simulink model "state_space_all_reduce_uio"  (R2018a)
settings: Solver=FixedStepAuto  StartTime=0.0  StopTime=3  FixedStep=tm  MaxStep=1e-4  RelTol=1e-5  AbsTol=1e-5
InitFcn:
  | SimulinkInit_linea_transmision
values from neighbouring files (symbols this model uses):
  b = 4.91    [SimulinkInit_linea_transmision.m]
  C = 1    [SimulinkInit_linea_transmision.m]
  C1 = 22e-6    (= 2.2e-05)    [SimulinkInit_linea_transmision.m]
  C2 = 22e-6    (= 2.2e-05)    [SimulinkInit_linea_transmision.m]
  C3 = 610e-6    (= 0.00061)    [SimulinkInit_linea_transmision.m]
  Cl = 20000e-6    (= 0.02)    [SimulinkInit_linea_transmision.m]
  Jd = 0.3    [SimulinkInit_linea_transmision.m]
  K = 25    [SimulinkInit_linea_transmision.m]    (also in uio_linear.m = K1+E*H)
  K1 = 9.66    [SimulinkInit_linea_transmision.m]    (also in uio_linear.m = K1')
  K11 = 0.8    [SimulinkInit_linea_transmision.m]
  K1d = 1.15    [SimulinkInit_linea_transmision.m]
  K2 = 6.97    [SimulinkInit_linea_transmision.m]
  K22 = 0.2    [SimulinkInit_linea_transmision.m]
  K2d = 1    [SimulinkInit_linea_transmision.m]
  K3 = 31.8    [SimulinkInit_linea_transmision.m]
  K33 = 0.23    [SimulinkInit_linea_transmision.m]
  K3d = 1    [SimulinkInit_linea_transmision.m]
  K4 = 15.1    [SimulinkInit_linea_transmision.m]
  Kd = 0.02    [SimulinkInit_linea_transmision.m]
  Kdc = 0.02    [SimulinkInit_linea_transmision.m]
  Kf = 1    [SimulinkInit_linea_transmision.m]
  Kh = 1.2    [SimulinkInit_linea_transmision.m]
  Ks = 21.5    [SimulinkInit_linea_transmision.m]
  Ksc = 3    [SimulinkInit_linea_transmision.m]
  Kv = 1    [SimulinkInit_linea_transmision.m]
  L = 5.2    [SimulinkInit_linea_transmision.m]
  L1 = 40e-3    (= 0.04)    [SimulinkInit_linea_transmision.m]
  L2 = 30e-3    (= 0.03)    [SimulinkInit_linea_transmision.m]
  L3 = 5e-3    (= 0.005)    [SimulinkInit_linea_transmision.m]
  L4 = 35e-6    (= 3.5e-05)    [SimulinkInit_linea_transmision.m]
  L5 = 22e-6    (= 2.2e-05)    [SimulinkInit_linea_transmision.m]
  L6 = 10e-6    (= 1e-05)    [SimulinkInit_linea_transmision.m]
  Pd = 0.1    [SimulinkInit_linea_transmision.m]
  R = 10    [SimulinkInit_linea_transmision.m]
  R1 = 0.1    [SimulinkInit_linea_transmision.m]
  R2 = 0.2    [SimulinkInit_linea_transmision.m]
  R3 = 1e-3    (= 0.001)    [SimulinkInit_linea_transmision.m]
  R4 = 0.005    [SimulinkInit_linea_transmision.m]
  R5 = 0.0012    [SimulinkInit_linea_transmision.m]
  R6 = 0.001    [SimulinkInit_linea_transmision.m]
  RL = 10    [SimulinkInit_linea_transmision.m]
  Sbin = 13.8    [SimulinkInit_linea_transmision.m]
  Svin = 2.91    [SimulinkInit_linea_transmision.m]
  T1 = 0.4    [SimulinkInit_linea_transmision.m]
  T2 = 1    [SimulinkInit_linea_transmision.m]
  T3 = 15    [SimulinkInit_linea_transmision.m]
  T4 = 2.5    [SimulinkInit_linea_transmision.m]
  Tao1d = 0.5    [SimulinkInit_linea_transmision.m]
  Tao2d = 0.125    [SimulinkInit_linea_transmision.m]
  Tcd = 0.2    [SimulinkInit_linea_transmision.m]
  Tcr = 0.01    [SimulinkInit_linea_transmision.m]
  Tf = 0.04    [SimulinkInit_linea_transmision.m]
  Tr = 950    [SimulinkInit_linea_transmision.m]
  Tt = 450    [SimulinkInit_linea_transmision.m]
  Ttd = 0.04    [SimulinkInit_linea_transmision.m]
  Tv = 0.05    [SimulinkInit_linea_transmision.m]
  V = 20    [SimulinkInit_linea_transmision.m]
  wref = 70000    [SimulinkInit_linea_transmision.m]
  X_acid = 1.2    [SimulinkInit_linea_transmision.m]
  X_meth = 0.35    [SimulinkInit_linea_transmision.m]
  Z = 3    [SimulinkInit_linea_transmision.m]
undefined symbols (not defined in the file or in its folder): Ad, ataque, Bd, c11, c12, c13, c14, C1o, c21, c22, c23, c24, C2o, c31, c32, c33, c34, C3o, c41, c42, c43, c44, C4o, Cd, F1, F2, F3, F4, H1, H2, H3, H4, K1U, K2U, K3U, K4U, T1s, T2s, T3s, T4s, T5s, tao1, tao2, taod, tm, uio1r, uio2r, uio3r, uio4r
libraries: neural x277, dsparch4 x4, powerlib_meascontrol x4, mpclib x1, simulink x1
(part 11 of 16)

== system state_space_all_reduce_uio/Function Fitting Neural Network2/Layer 2/Delays 1 ==
  "p{2}" : Inport  PortDimensions=30  SampleTime=4e-05
      mask Display: e = 0.06;c1 = [120 230 180]/255;c2 = ([120 230 180]+0)/(256+128);c3 = ([120 230 180]+128)/(256+128);patch([0 1 1 0],[0 0 1 1],c1);patch([0 1 1 1-e 1-e 0+e],[0 0 1 1-e 0+e 0+e],c2);patch([0 0 1 1-e 0+e 0+e],[0 1 1 1-e 1-e 0+e],c3);plot([0 1 1 0 0],[0 0 1 1 0]);
  mux : Mux  Inputs=1
      mask Display: e = 0.06;c1 = [120 150 230]/255;c2 = ([120 150 230]+0)/383;c3 = ([120 150 230]+128)/383;patch([0 1 1 0],[0 0 1 1],c1);patch([0 1 1 1-e 1-e 0+e],[0 0 1 1-e 0+e 0+e],c2);patch([0 0 1 1-e 0+e 0+e],[0 1 1 1-e 1-e 0+e],c3);plot([0 1 1 0 0],[0 0 1 1 0]);disp('Mux')
  "pd{2,1}" : Outport
      mask Display: e = 0.06;c1 = [120 230 180]/255;c2 = ([120 230 180]+0)/(256+128);c3 = ([120 230 180]+128)/(256+128);patch([0 1 1 0],[0 0 1 1],c1);patch([0 1 1 1-e 1-e 0+e],[0 0 1 1-e 0+e 0+e],c2);patch([0 0 1 1-e 0+e 0+e],[0 1 1 1-e 1-e 0+e],c3);plot([0 1 1 0 0],[0 0 1 1 0]);
  wires:
  "p{2}"/1 -> mux/1
  mux/1 -> "pd{2,1}"/1

== system state_space_all_reduce_uio/Function Fitting Neural Network2/Layer 2/LW{2,1} ==
  "ad{2,1}" : Inport  PortDimensions=30  SampleTime=4e-05
      mask Display: e = 0.06;c1 = [120 230 180]/255;c2 = ([120 230 180]+0)/(256+128);c3 = ([120 230 180]+128)/(256+128);patch([0 1 1 0],[0 0 1 1],c1);patch([0 1 1 1-e 1-e 0+e],[0 0 1 1-e 0+e 0+e],c2);patch([0 0 1 1-e 0+e 0+e],[0 1 1 1-e 1-e 0+e],c3);plot([0 1 1 0 0],[0 0 1 1 0]);
  "IW{2,1}(1,:)'" : Constant  Value=[0.0184375105713764954329381140496479929424822330474853515625;-0.3207474044058853390737340305349789559841156005859375;-0.258723890615078444543684099699021317064762115478515625;0.317168024231023137904372788398177362978458404541015625;-0.2348184046563489280057268615564680658280849456787109375;-0.255707110628516309791535832118825055658817291259765625;0.296343028954519638329401232113013975322246551513671875;0.371965104778058164303189414567896164953708648681640625;-0.2125065463660006093160603768410510383546352386474609375;-0.034179812701825962317769835863145999610424041748046875;-0.057864679635199166296555262078982195816934108734130859375;-0.351082171280389154777168414511834271252155303955078125;-0.3249901438598581382422025853884406387805938720703125;-0.65104176452594775259541393097606487572193145751953125;0.431202379857678230745676728474791161715984344482421875;-0.2121306307099686538908400734726455993950366973876953125;-0.06308824296903732531394126681334455497562885284423828125;0.367066697908505601422035624636919237673282623291015625;0.01518189243024294955708430876484271720983088016510009765625;0.32625866653337265432810454512946307659149169921875;0.0885035086889276179089591778392787091434001922607421875;-0.2141364027072355791236901723095797933638095855712890625;0.306630144040333119104246861752471886575222015380859375;-0.36178542478347919253423015106818638741970062255859375;0.16713066534734088985914013392175547778606414794921875;0.080764762392429745307964594758232124149799346923828125;-0.09468771758867734755771294885562383569777011871337890625;0.275883830902875992752143474717740900814533233642578125;-0.05263790406327938098396401755962870083749294281005859375;-0.289428356624796434548585466473014093935489654541015625]
      mask Display: e = 0.06;c1 = [120 150 230]/255;c2 = ([120 150 230]+0)/383;c3 = ([120 150 230]+128)/383;patch([0 1 1 0],[0 0 1 1],c1);patch([0 1 1 1-e 1-e 0+e],[0 0 1 1-e 0+e 0+e],c2);patch([0 0 1 1-e 0+e 0+e],[0 1 1 1-e 1-e 0+e],c3);plot([0 1 1 0 0],[0 0 1 1 0]);disp('weights');
  "IW{2,1}(10,:)'" : Constant  Value=[0.25213999606592774060942474534385837614536285400390625;-0.14455762474562006136835634606541134417057037353515625;-0.06961510156886237254969529431036789901554584503173828125;0.1603737673638012950494413644264568574726581573486328125;-0.305341118440620895579939997332985512912273406982421875;-0.1785844871078878792758359850267879664897918701171875;-0.388367504053590051338318289708695374429225921630859375;0.28604588230512273394623434796812944114208221435546875;-0.2399829384761393014091623854255885817110538482666015625;-0.3128381144117107215407713738386519253253936767578125;-0.09330072155796391430992997584326076321303844451904296875;-0.215158223537697923521960774451144970953464508056640625;-0.50092245439516636107413205536431632936000823974609375;-0.2070651195794658006033017727531841956079006195068359375;-0.409070713649272221790198500457336194813251495361328125;0.0693704580088942146520736287129693664610385894775390625;-0.30869209327984925561594309328938834369182586669921875;-0.32515187820802504692352385973208583891391754150390625;0.016466106698614375869471615487782401032745838165283203125;-0.2276231422022782224789949623300344683229923248291015625;-0.33567427593388943218855047234683297574520111083984375;-0.12189318592657509554566530596275697462260723114013671875;-0.158401987289081225274145481307641603052616119384765625;0.327150254991547428939924202495603822171688079833984375;-0.01114075490773060346516576402109421906061470508575439453125;0.34095259387459642130835391071741469204425811767578125;-0.2760674175692054976849476588540710508823394775390625;0.469496337468091440303652461807359941303730010986328125;0.132054144394454897604163079449790529906749725341796875;0.428690959612985589277656117701553739607334136962890625]
      mask Display: e = 0.06;c1 = [120 150 230]/255;c2 = ([120 150 230]+0)/383;c3 = ([120 150 230]+128)/383;patch([0 1 1 0],[0 0 1 1],c1);patch([0 1 1 1-e 1-e 0+e],[0 0 1 1-e 0+e 0+e],c2);patch([0 0 1 1-e 0+e 0+e],[0 1 1 1-e 1-e 0+e],c3);plot([0 1 1 0 0],[0 0 1 1 0]);disp('weights');
  "IW{2,1}(2,:)'" : Constant  Value=[0.041585503274869810297342809235487948171794414520263671875;0.11544137404087850828915406964370049536228179931640625;0.349065779270401943534807287505827844142913818359375;-0.40931464495936664693687134786159731447696685791015625;-0.00783113330299452237159840706226532347500324249267578125;-0.0193261270553777807224005158559521078132092952728271484375;0.077000005947650718152175386421731673181056976318359375;0.4194517105169193182945264197769574820995330810546875;-0.09417134110736848084943773073973716236650943756103515625;-0.168175625372271542179447578746476210653781890869140625;-0.232558522736353523452379477021167986094951629638671875;-0.1797983512845484355135994292140821926295757293701171875;-0.379140710743090247891728949980461038649082183837890625;0.377741239559755970223164922572323121130466461181640625;-0.1326415588656811028744897384967771358788013458251953125;-0.5352894650767250350753556631389074027538299560546875;0.297691104134658102164934234679094515740871429443359375;0.0237853849170003017743368900482892058789730072021484375;-0.052964121508768509383191513961719465442001819610595703125;0.306316490100252580841555527513264678418636322021484375;-0.260822681627116803593224858559551648795604705810546875;-0.1891507767148402352486158406463800929486751556396484375;0.311638174833818337727819880456081591546535491943359375;0.1356072046945252795868697148762294091284275054931640625;0.400986861647478709524961004717624746263027191162109375;0.38378342432170853282258349281619302928447723388671875;-0.448721101092427743228796543917269445955753326416015625;0.0864458793766731681262882602823083288967609405517578125;-0.52143010488950081171566353077651001513004302978515625;-0.048545477186974543559738748399468022398650646209716796875]
      mask Display: e = 0.06;c1 = [120 150 230]/255;c2 = ([120 150 230]+0)/383;c3 = ([120 150 230]+128)/383;patch([0 1 1 0],[0 0 1 1],c1);patch([0 1 1 1-e 1-e 0+e],[0 0 1 1-e 0+e 0+e],c2);patch([0 0 1 1-e 0+e 0+e],[0 1 1 1-e 1-e 0+e],c3);plot([0 1 1 0 0],[0 0 1 1 0]);disp('weights');
  "IW{2,1}(3,:)'" : Constant  Value=[0.230049474251456220752487524805474095046520233154296875;-0.1916684540517501200707073394369217567145824432373046875;-0.043065521108052569332347303543429006822407245635986328125;0.4112236894534666564737790395156480371952056884765625;-0.1846368980317161512250123678313684649765491485595703125;0.42433664741991050650682382183731533586978912353515625;-0.023505964392957261199779139815291273407638072967529296875;-0.09776584761341385043653673392327618785202503204345703125;-0.335510895415650767237281115740188397467136383056640625;-0.371898630629495574595466678147204220294952392578125;-0.327186967840456033318474737825454212725162506103515625;0.0238201757398892322026284773528459481894969940185546875;0.00986592894299041962835605801274141413159668445587158203125;0.38288250104145371555119936601840890944004058837890625;-0.2336284020105205694317618281274917535483837127685546875;0.055488276848311979261296755794319324195384979248046875;-0.33142109618668380566219866523169912397861480712890625;0.140990365099240844148908990973723120987415313720703125;0.2056025990494126653995721198953106068074703216552734375;-0.34378739105746680682074156720773316919803619384765625;-0.26957922713858983865264917767490260303020477294921875;0.0854406576220511360109099996407167054712772369384765625;0.1527916152213713851804044452364905737340450286865234375;0.041593124777035618555576235166881815530359745025634765625;-0.1579944403086087911791679516682052053511142730712890625;0.09263578756269563729830451848101802170276641845703125;-0.208438235923540216010252379419398494064807891845703125;0.06451475639070035350552956288083805702626705169677734375;0.16796927963178642784214389394037425518035888671875;0.339285277243822458448363477145903743803501129150390625]
      mask Display: e = 0.06;c1 = [120 150 230]/255;c2 = ([120 150 230]+0)/383;c3 = ([120 150 230]+128)/383;patch([0 1 1 0],[0 0 1 1],c1);patch([0 1 1 1-e 1-e 0+e],[0 0 1 1-e 0+e 0+e],c2);patch([0 0 1 1-e 0+e 0+e],[0 1 1 1-e 1-e 0+e],c3);plot([0 1 1 0 0],[0 0 1 1 0]);disp('weights');
  "IW{2,1}(4,:)'" : Constant  Value=[-0.336431789441323403355710297546465881168842315673828125;-0.1978097242838057212566127418540418148040771484375;0.0540585346863775573211796654504723846912384033203125;0.2401411533138659015751414926853612996637821197509765625;-0.152055759398248502289874295456684194505214691162109375;-0.0161008429425668897483348018795368261635303497314453125;-0.629549467732146705856166590820066630840301513671875;-0.39304263686412876932507742822053842246532440185546875;0.161331262566255961843353361473418772220611572265625;0.2244920641490608381740656795955146662890911102294921875;0.5677832049493414245944222784601151943206787109375;-0.42045819204395062929080495450762100517749786376953125;0.299008296283185870390042282451759092509746551513671875;-0.1564468875344843523667037743507535196840763092041015625;-0.1740896721119109258335555523444782011210918426513671875;0.0897368283863136662059645232147886417806148529052734375;-0.26818537372390360840057610403164289891719818115234375;-0.11729170340152694773649955095606856048107147216796875;0.31727665098534629795068440216709859669208526611328125;0.08358180532877455826135104643981321714818477630615234375;0.21917514442586971679105545263155363500118255615234375;0.3272449904986991509048266379977576434612274169921875;-0.0906465471486596341410546529004932381212711334228515625;0.30481314245177515420692770931054838001728057861328125;0.267122982877820602798379923115135170519351959228515625;-0.22117562226847475859159430910949595272541046142578125;-0.283805758176242040047299042271333746612071990966796875;-0.0948060837770212383457391069896402768790721893310546875;-0.471164491708904009659164557888288982212543487548828125;-0.348997982084099656052700311192893423140048980712890625]
      mask Display: e = 0.06;c1 = [120 150 230]/255;c2 = ([120 150 230]+0)/383;c3 = ([120 150 230]+128)/383;patch([0 1 1 0],[0 0 1 1],c1);patch([0 1 1 1-e 1-e 0+e],[0 0 1 1-e 0+e 0+e],c2);patch([0 0 1 1-e 0+e 0+e],[0 1 1 1-e 1-e 0+e],c3);plot([0 1 1 0 0],[0 0 1 1 0]);disp('weights');
  "IW{2,1}(5,:)'" : Constant  Value=[0.164688299442875829559085332221002317965030670166015625;0.10785250831244030944588985221344046294689178466796875;-0.15404601317541521954268546323874033987522125244140625;-0.1628537357754085423966472490064916200935840606689453125;-0.150705373392541031041247379107517190277576446533203125;0.265264795415320275839832220299285836517810821533203125;-0.2350142100681567314257591760906507261097431182861328125;-0.250460541594123953235140334072639234364032745361328125;0.1461604812968614053314553302698186598718166351318359375;0.2514439304293769605891384344431571662425994873046875;0.0861604042127249447613479560459381900727748870849609375;-0.1302580078716808198446841515760752372443675994873046875;-0.327253374220396853200298892261344008147716522216796875;0.349204696823601778987722354941070079803466796875;0.0360425736598270762822693313864874653518199920654296875;0.2407252925848043234591244754483341239392757415771484375;0.04406903635090701765175680293395998887717723846435546875;-0.0036160370528572987301740848664621807984076440334320068359375;-0.49636954282977097108187081175856292247772216796875;0.351573928050453066163072435301728546619415283203125;0.25107458623996647961718053920776583254337310791015625;-0.0023535595687285935928567681685308343730866909027099609375;0.316123158478801735693508589974953792989253997802734375;-0.2433328742218157092480623759911395609378814697265625;-0.4122692805971350793470264761708676815032958984375;0.35479759458358028911817427797359414398670196533203125;-0.4299111239151687247073141406872309744358062744140625;-0.211466103498746560429566443417570553719997406005859375;-0.3485846833605690253676812062622047960758209228515625;-0.472508218100085031210255692712962627410888671875]
      mask Display: e = 0.06;c1 = [120 150 230]/255;c2 = ([120 150 230]+0)/383;c3 = ([120 150 230]+128)/383;patch([0 1 1 0],[0 0 1 1],c1);patch([0 1 1 1-e 1-e 0+e],[0 0 1 1-e 0+e 0+e],c2);patch([0 0 1 1-e 0+e 0+e],[0 1 1 1-e 1-e 0+e],c3);plot([0 1 1 0 0],[0 0 1 1 0]);disp('weights');
  "IW{2,1}(6,:)'" : Constant  Value=[0.42542774037770614281583902993588708341121673583984375;0.1806126895096568374388112943051964975893497467041015625;0.10990035257033602122955784352598129771649837493896484375;-0.2039703371170145940194373679332784377038478851318359375;0.41935713871300295263466750839143060147762298583984375;-0.298890464705078684470862526723067276179790496826171875;-0.2365188454277212526388751712147495709359645843505859375;0.365337724342684799783143034801469184458255767822265625;0.1547993776321235637194462242405279539525508880615234375;0.2028271506292016190808880082840914838016033172607421875;-0.380179147430922903527772405141149647533893585205078125;0.2682905216015558647058014685171656310558319091796875;-0.2619162668797319071245510713197290897369384765625;0.04785079468079100895039346141857095062732696533203125;-0.30607965595790498358752529384219087660312652587890625;-0.006878514311119412853734456092524851555936038494110107421875;0.434070987765542926073436547085293568670749664306640625;0.1404433798536896815800645299532334320247173309326171875;0.151759774102104894044629190830164588987827301025390625;0.373701433100081248372958953041234053671360015869140625;-0.277597077745849130092636869449052028357982635498046875;0.08677371205675876719709549433900974690914154052734375;0.2039772429519299823397204818320460617542266845703125;0.001308243964541404812107483479621805599890649318695068359375;-0.1429804709159524234163285427712253294885158538818359375;0.457197721872434625911552075194776989519596099853515625;-0.25082580264625631283337270360789261758327484130859375;-0.38702427147571227816769123819540254771709442138671875;-0.32912256252535510014922692789696156978607177734375;-0.36374059657364188336003962831455282866954803466796875]
      mask Display: e = 0.06;c1 = [120 150 230]/255;c2 = ([120 150 230]+0)/383;c3 = ([120 150 230]+128)/383;patch([0 1 1 0],[0 0 1 1],c1);patch([0 1 1 1-e 1-e 0+e],[0 0 1 1-e 0+e 0+e],c2);patch([0 0 1 1-e 0+e 0+e],[0 1 1 1-e 1-e 0+e],c3);plot([0 1 1 0 0],[0 0 1 1 0]);disp('weights');
  "IW{2,1}(7,:)'" : Constant  Value=[-0.057516131246669162380147355406734277494251728057861328125;0.2135251843622437417646864332709810696542263031005859375;0.27246734386235627045635965259862132370471954345703125;0.254515790201969405170956406436744146049022674560546875;-0.1698633391815599080754140004501095972955226898193359375;-0.2086958942668961369815150419526617042720317840576171875;-0.133263892552788199008517722177202813327312469482421875;0.2880970181078044145550620669382624328136444091796875;0.09478415823026896391834128507980494759976863861083984375;-0.2954632893039261798406869274913333356380462646484375;0.2268666564800077833918834357973537407815456390380859375;0.3795654541896624767360890473355539143085479736328125;0.16738148476050807023085553737473674118518829345703125;0.134153163956483079122250501313828863203525543212890625;-0.10909619087766632417046963610118837095797061920166015625;-0.03261780278571511926255510616101673804223537445068359375;0.25269060559296685486430078526609577238559722900390625;0.371997168912341080737604670503060333430767059326171875;-0.367326041482953502548269852923112921416759490966796875;-0.40404697312835546885168014341616071760654449462890625;0.11466396342484046211307457951988908462226390838623046875;-0.1922989559856618513311588003489305265247821807861328125;0.025984316880847894981609869091698783449828624725341796875;0.14356667876398343519639411169919185340404510498046875;0.33922025107628128726133809323073364794254302978515625;0.355012087308320067879918724429444409906864166259765625;-0.426157360218916425598223440829315222799777984619140625;0.33455559200657958296432070710579864680767059326171875;0.4125704492923691901751226396299898624420166015625;-0.099273006662906893016184994849027134478092193603515625]
      mask Display: e = 0.06;c1 = [120 150 230]/255;c2 = ([120 150 230]+0)/383;c3 = ([120 150 230]+128)/383;patch([0 1 1 0],[0 0 1 1],c1);patch([0 1 1 1-e 1-e 0+e],[0 0 1 1-e 0+e 0+e],c2);patch([0 0 1 1-e 0+e 0+e],[0 1 1 1-e 1-e 0+e],c3);plot([0 1 1 0 0],[0 0 1 1 0]);disp('weights');
  "IW{2,1}(8,:)'" : Constant  Value=[0.357557120957959051477104139848961494863033294677734375;-0.324928633542516720478232628011028282344341278076171875;-0.07930516037086297875813301061498350463807582855224609375;-0.28874199505402298182588083363953046500682830810546875;-0.2516472588370939345026044975384138524532318115234375;-0.010042619754616378957567945917617180384695529937744140625;0.2145751450180266306499987649658578447997570037841796875;0.210624859953667920020592418950400315225124359130859375;-0.3373781774752988571464129563537426292896270751953125;0.12287871074119126324486472867647535167634487152099609375;-0.449194677729232216822907730602310039103031158447265625;0.05904983123335334760373172002800856716930866241455078125;-0.4077680319699281685785763329477049410343170166015625;0.27516524196255398582167117638164199888706207275390625;0.190403598242514959792970330454409122467041015625;-0.2261855081420083291021683180588297545909881591796875;-0.1937395034234277446660854593574185855686664581298828125;-0.319164431923269376056850887835025787353515625;0.469226904619882756453108640926075167953968048095703125;0.14841293832629798288280653650872409343719482421875;0.055704462912061540602604026162225636653602123260498046875;0.1903900399586629654802294453475042246282100677490234375;0.156720369210245069613307578038075007498264312744140625;0.207598846074474818745869697522721253335475921630859375;-0.2380687019027708239971019565928145311772823333740234375;-0.396145205707853442778088037812267430126667022705078125;-0.0024840294984183369959851450659016336430795490741729736328125;-0.0283736624331737928572660933923543780110776424407958984375;0.3981593678783355017003486864268779754638671875;-0.40024971812002563265053822760819457471370697021484375]
      mask Display: e = 0.06;c1 = [120 150 230]/255;c2 = ([120 150 230]+0)/383;c3 = ([120 150 230]+128)/383;patch([0 1 1 0],[0 0 1 1],c1);patch([0 1 1 1-e 1-e 0+e],[0 0 1 1-e 0+e 0+e],c2);patch([0 0 1 1-e 0+e 0+e],[0 1 1 1-e 1-e 0+e],c3);plot([0 1 1 0 0],[0 0 1 1 0]);disp('weights');
  "IW{2,1}(9,:)'" : Constant  Value=[0.15663266180138124550325073869316838681697845458984375;-0.1821711882840743312872433534721494652330875396728515625;-0.280604972191765000832930354590644128620624542236328125;0.0143041068744069917173522554776354809291660785675048828125;0.40102692467406086951342558677424676716327667236328125;0.303645890492979464436729131193715147674083709716796875;0.164927158966075293466957418786478228867053985595703125;-0.25989400727902889354226090290467254817485809326171875;0.147889168715451269076055496043409220874309539794921875;-0.041574157283416672548082004823299939744174480438232421875;0.406086131207421541233770767576061189174652099609375;0.4191847569567201947648982240934856235980987548828125;0.371084597522654158208155195097788237035274505615234375;-0.489610292428150517540785813253023661673069000244140625;0.3429172437621594848877748518134467303752899169921875;0.1288859989504568537288520246875123120844364166259765625;0.1733123812465842961128004162674187682569026947021484375;0.269390498789371990451257943277596496045589447021484375;-0.1864825303322950877937813629614538513123989105224609375;-0.271169445852704971144930823356844484806060791015625;0.2700039189624983126947199707501567900180816650390625;-0.2207635892170148050883682344647240824997425079345703125;0.0719184616146260058400230263941921293735504150390625;0.1368431140769651166433362732277601025998592376708984375;0.003787976087533020085051926884034401155076920986175537109375;0.380566442447093533640867235590121708810329437255859375;-0.214194279564747791511081231874413788318634033203125;-0.09287307859184086578085981500407797284424304962158203125;-0.4522135567590497284840012071072123944759368896484375;0.2645955661652166224229176805238239467144012451171875]
      mask Display: e = 0.06;c1 = [120 150 230]/255;c2 = ([120 150 230]+0)/383;c3 = ([120 150 230]+128)/383;patch([0 1 1 0],[0 0 1 1],c1);patch([0 1 1 1-e 1-e 0+e],[0 0 1 1-e 0+e 0+e],c2);patch([0 0 1 1-e 0+e 0+e],[0 1 1 1-e 1-e 0+e],c3);plot([0 1 1 0 0],[0 0 1 1 0]);disp('weights');
  Mux : Mux  Inputs=10
      mask Display: e = 0.06;c1 = [120 150 230]/255;c2 = ([120 150 230]+0)/383;c3 = ([120 150 230]+128)/383;patch([0 1 1 0],[0 0 1 1],c1);patch([0 1 1 1-e 1-e 0+e],[0 0 1 1-e 0+e 0+e],c2);patch([0 0 1 1-e 0+e 0+e],[0 1 1 1-e 1-e 0+e],c3);plot([0 1 1 0 0],[0 0 1 1 0]);disp('Mux');
  dotprod{1..10} (10 alike) : neural/Weight Functions/dotprod
  "lz{2,1}" : Outport
      mask Display: e = 0.06;c1 = [120 230 180]/255;c2 = ([120 230 180]+0)/(256+128);c3 = ([120 230 180]+128)/(256+128);patch([0 1 1 0],[0 0 1 1],c1);patch([0 1 1 1-e 1-e 0+e],[0 0 1 1-e 0+e 0+e],c2);patch([0 0 1 1-e 0+e 0+e],[0 1 1 1-e 1-e 0+e],c3);plot([0 1 1 0 0],[0 0 1 1 0]);
  wires:
  "IW{2,1}(1,:)'"/1 -> dotprod1/1
  "ad{2,1}"/1 -> dotprod1/2, dotprod2/2, dotprod3/2, dotprod4/2, dotprod5/2, dotprod6/2, dotprod7/2, dotprod8/2, dotprod9/2, dotprod10/2
  dotprod1/1 -> Mux/1
  "IW{2,1}(2,:)'"/1 -> dotprod2/1
  dotprod2/1 -> Mux/2
  "IW{2,1}(3,:)'"/1 -> dotprod3/1
  dotprod3/1 -> Mux/3
  "IW{2,1}(4,:)'"/1 -> dotprod4/1
  dotprod4/1 -> Mux/4
  "IW{2,1}(5,:)'"/1 -> dotprod5/1
  dotprod5/1 -> Mux/5
  "IW{2,1}(6,:)'"/1 -> dotprod6/1
  dotprod6/1 -> Mux/6
  "IW{2,1}(7,:)'"/1 -> dotprod7/1
  dotprod7/1 -> Mux/7
  "IW{2,1}(8,:)'"/1 -> dotprod8/1
  dotprod8/1 -> Mux/8
  "IW{2,1}(9,:)'"/1 -> dotprod9/1
  dotprod9/1 -> Mux/9
  "IW{2,1}(10,:)'"/1 -> dotprod10/1
  dotprod10/1 -> Mux/10
  Mux/1 -> "lz{2,1}"/1

== system state_space_all_reduce_uio/Function Fitting Neural Network2/Layer 3/Delays 1 ==
  "p{3}" : Inport  PortDimensions=10  SampleTime=4e-05
      mask Display: e = 0.06;c1 = [120 230 180]/255;c2 = ([120 230 180]+0)/(256+128);c3 = ([120 230 180]+128)/(256+128);patch([0 1 1 0],[0 0 1 1],c1);patch([0 1 1 1-e 1-e 0+e],[0 0 1 1-e 0+e 0+e],c2);patch([0 0 1 1-e 0+e 0+e],[0 1 1 1-e 1-e 0+e],c3);plot([0 1 1 0 0],[0 0 1 1 0]);
  mux : Mux  Inputs=1
      mask Display: e = 0.06;c1 = [120 150 230]/255;c2 = ([120 150 230]+0)/383;c3 = ([120 150 230]+128)/383;patch([0 1 1 0],[0 0 1 1],c1);patch([0 1 1 1-e 1-e 0+e],[0 0 1 1-e 0+e 0+e],c2);patch([0 0 1 1-e 0+e 0+e],[0 1 1 1-e 1-e 0+e],c3);plot([0 1 1 0 0],[0 0 1 1 0]);disp('Mux')
  "pd{3,2}" : Outport
      mask Display: e = 0.06;c1 = [120 230 180]/255;c2 = ([120 230 180]+0)/(256+128);c3 = ([120 230 180]+128)/(256+128);patch([0 1 1 0],[0 0 1 1],c1);patch([0 1 1 1-e 1-e 0+e],[0 0 1 1-e 0+e 0+e],c2);patch([0 0 1 1-e 0+e 0+e],[0 1 1 1-e 1-e 0+e],c3);plot([0 1 1 0 0],[0 0 1 1 0]);
  wires:
  "p{3}"/1 -> mux/1
  mux/1 -> "pd{3,2}"/1

== system state_space_all_reduce_uio/Function Fitting Neural Network2/Layer 3/LW{3,2} ==
  "ad{3,2}" : Inport  PortDimensions=10  SampleTime=4e-05
      mask Display: e = 0.06;c1 = [120 230 180]/255;c2 = ([120 230 180]+0)/(256+128);c3 = ([120 230 180]+128)/(256+128);patch([0 1 1 0],[0 0 1 1],c1);patch([0 1 1 1-e 1-e 0+e],[0 0 1 1-e 0+e 0+e],c2);patch([0 0 1 1-e 0+e 0+e],[0 1 1 1-e 1-e 0+e],c3);plot([0 1 1 0 0],[0 0 1 1 0]);
  "IW{3,2}(1,:)'" : Constant  Value=[-0.5468759942672447582623362904996611177921295166015625;0.1770317650502955253433157167819445021450519561767578125;-0.056466388283832373573556395740524749271571636199951171875;0.7027027426868939219417597996653057634830474853515625;-0.06064628236359957680345900143947801552712917327880859375;0.9090180903427065306487975249183364212512969970703125;-0.7259630189879360262494856215198524296283721923828125;-0.67866271606338435251615237575606442987918853759765625;-0.327925619562051517963396918275975622236728668212890625;-0.43619437688946194331407468780525960028171539306640625]
      mask Display: e = 0.06;c1 = [120 150 230]/255;c2 = ([120 150 230]+0)/383;c3 = ([120 150 230]+128)/383;patch([0 1 1 0],[0 0 1 1],c1);patch([0 1 1 1-e 1-e 0+e],[0 0 1 1-e 0+e 0+e],c2);patch([0 0 1 1-e 0+e 0+e],[0 1 1 1-e 1-e 0+e],c3);plot([0 1 1 0 0],[0 0 1 1 0]);disp('weights');
  "IW{3,2}(10,:)'" : Constant  Value=[-0.93689507813734029806340686263865791261196136474609375;-0.208500694373201955755803282954730093479156494140625;0.384946764990786949311996067990548908710479736328125;-0.1986132154486971723716948190485709346830844879150390625;-0.327237447269842107733239799927105195820331573486328125;0.18340575001850722980378805004875175654888153076171875;0.61115242648222156685022810052032582461833953857421875;0.95054089273608755039646212026127614080905914306640625;-0.38134574986875635627114888848154805600643157958984375;0.02990330111657067690966727013801573775708675384521484375]
      mask Display: e = 0.06;c1 = [120 150 230]/255;c2 = ([120 150 230]+0)/383;c3 = ([120 150 230]+128)/383;patch([0 1 1 0],[0 0 1 1],c1);patch([0 1 1 1-e 1-e 0+e],[0 0 1 1-e 0+e 0+e],c2);patch([0 0 1 1-e 0+e 0+e],[0 1 1 1-e 1-e 0+e],c3);plot([0 1 1 0 0],[0 0 1 1 0]);disp('weights');
  "IW{3,2}(2,:)'" : Constant  Value=[-0.709204036597272935438240892835892736911773681640625;-0.156729362649643710891922410155530087649822235107421875;0.85180690635675826438699687059852294623851776123046875;0.029468232796269477891115684542455710470676422119140625;-0.425388880494024401723862638391437940299510955810546875;-0.81280425361824837349189465385279618203639984130859375;0.482049224382242569308942847783328033983707427978515625;0.40150930826275710305850452641607262194156646728515625;-0.58799599491496457037698064596042968332767486572265625;0.360066901966373087429218458055402152240276336669921875]
      mask Display: e = 0.06;c1 = [120 150 230]/255;c2 = ([120 150 230]+0)/383;c3 = ([120 150 230]+128)/383;patch([0 1 1 0],[0 0 1 1],c1);patch([0 1 1 1-e 1-e 0+e],[0 0 1 1-e 0+e 0+e],c2);patch([0 0 1 1-e 0+e 0+e],[0 1 1 1-e 1-e 0+e],c3);plot([0 1 1 0 0],[0 0 1 1 0]);disp('weights');
  "IW{3,2}(3,:)'" : Constant  Value=[0.6391947626131029291940421899198554456233978271484375;-0.1455325020145506742519359022480784915387630462646484375;0.7878650121670889294733797214576043188571929931640625;-0.8306656631185720396359783990192227065563201904296875;-0.189024195312362142118445262894965708255767822265625;0.40596636991776391401032242356450296938419342041015625;-0.58709492691347253678912920804577879607677459716796875;-0.356316877137873799785694473030162043869495391845703125;-0.792027254318413032052603739430196583271026611328125;-0.205214397052488284334259560637292452156543731689453125]
      mask Display: e = 0.06;c1 = [120 150 230]/255;c2 = ([120 150 230]+0)/383;c3 = ([120 150 230]+128)/383;patch([0 1 1 0],[0 0 1 1],c1);patch([0 1 1 1-e 1-e 0+e],[0 0 1 1-e 0+e 0+e],c2);patch([0 0 1 1-e 0+e 0+e],[0 1 1 1-e 1-e 0+e],c3);plot([0 1 1 0 0],[0 0 1 1 0]);disp('weights');
  "IW{3,2}(4,:)'" : Constant  Value=[0.8888969058457496519309870564029552042484283447265625;0.35641791851674120561455083588953129947185516357421875;0.97228824655911838537036828711279667913913726806640625;0.539075874482534356246787865529768168926239013671875;-0.2396894186908370694144565504757338203489780426025390625;-0.95551731627037572724958636172232218086719512939453125;-0.7048482321662012939356145579949952661991119384765625;0.09635570839727129743845779330513323657214641571044921875;-0.08537862058117580421612302643552538938820362091064453125;-0.159130374572028665536294056437327526509761810302734375]
      mask Display: e = 0.06;c1 = [120 150 230]/255;c2 = ([120 150 230]+0)/383;c3 = ([120 150 230]+128)/383;patch([0 1 1 0],[0 0 1 1],c1);patch([0 1 1 1-e 1-e 0+e],[0 0 1 1-e 0+e 0+e],c2);patch([0 0 1 1-e 0+e 0+e],[0 1 1 1-e 1-e 0+e],c3);plot([0 1 1 0 0],[0 0 1 1 0]);disp('weights');
  "IW{3,2}(5,:)'" : Constant  Value=[0.6240759653480141277981374514638446271419525146484375;-0.12825199107295193190481086276122368872165679931640625;0.1460466301033048475144227040800615213811397552490234375;0.554715066133085077382247618515975773334503173828125;0.442708002808997080901320941848098300397396087646484375;-1.055542206976529673312370505300350487232208251953125;0.152486997266370327697160291791078634560108184814453125;0.2055736559127920026757152527352445758879184722900390625;-0.131952756588289921158008155543939210474491119384765625;-0.99103455781794969059461664073751308023929595947265625]
      mask Display: e = 0.06;c1 = [120 150 230]/255;c2 = ([120 150 230]+0)/383;c3 = ([120 150 230]+128)/383;patch([0 1 1 0],[0 0 1 1],c1);patch([0 1 1 1-e 1-e 0+e],[0 0 1 1-e 0+e 0+e],c2);patch([0 0 1 1-e 0+e 0+e],[0 1 1 1-e 1-e 0+e],c3);plot([0 1 1 0 0],[0 0 1 1 0]);disp('weights');
  "IW{3,2}(6,:)'" : Constant  Value=[0.3616307727597594112722845238749869167804718017578125;-0.60065801034336019359471947609563358128070831298828125;0.3345920080974018606667641506646759808063507080078125;0.97663511645704870201001313034794293344020843505859375;-0.197838473709368523056895128320320509374141693115234375;-0.56033422849399350251786700027878396213054656982421875;0.5691960117092411675088214906281791627407073974609375;0.1915915848444667834993282440336770378053188323974609375;0.63152744125053195123342675287858583033084869384765625;0.327150173323405291103682657194440253078937530517578125]
      mask Display: e = 0.06;c1 = [120 150 230]/255;c2 = ([120 150 230]+0)/383;c3 = ([120 150 230]+128)/383;patch([0 1 1 0],[0 0 1 1],c1);patch([0 1 1 1-e 1-e 0+e],[0 0 1 1-e 0+e 0+e],c2);patch([0 0 1 1-e 0+e 0+e],[0 1 1 1-e 1-e 0+e],c3);plot([0 1 1 0 0],[0 0 1 1 0]);disp('weights');
  "IW{3,2}(7,:)'" : Constant  Value=[-0.333624521764894821362901211614371277391910552978515625;0.48572241492961987230359000022872351109981536865234375;0.28741745295952458860710976296104490756988525390625;0.69611915113931266407831799369887448847293853759765625;0.250308451516423613458783847818267531692981719970703125;-0.464309768043250470359595283298403955996036529541015625;-0.09694389533437959560746577380996313877403736114501953125;1.297032771287094821133223376818932592868804931640625;0.04402660979404791896651971683240844868123531341552734375;0.55835682331147362678080980913364328444004058837890625]
      mask Display: e = 0.06;c1 = [120 150 230]/255;c2 = ([120 150 230]+0)/383;c3 = ([120 150 230]+128)/383;patch([0 1 1 0],[0 0 1 1],c1);patch([0 1 1 1-e 1-e 0+e],[0 0 1 1-e 0+e 0+e],c2);patch([0 0 1 1-e 0+e 0+e],[0 1 1 1-e 1-e 0+e],c3);plot([0 1 1 0 0],[0 0 1 1 0]);disp('weights');
  "IW{3,2}(8,:)'" : Constant  Value=[0.33813056585878487059204644538112916052341461181640625;-0.06348322237866547979034947957188705913722515106201171875;0.44847109001946183770570542037603445351123809814453125;-0.5222135281230839698451973163173533976078033447265625;0.38702707118188595103447369183413684368133544921875;0.5719688731611862753112518475973047316074371337890625;-0.78992582295522850710511875149677507579326629638671875;0.2049774458226645557079592663285438902676105499267578125;-0.103987628536826637315471089095808565616607666015625;-0.9466154426447423997359464920009486377239227294921875]
      mask Display: e = 0.06;c1 = [120 150 230]/255;c2 = ([120 150 230]+0)/383;c3 = ([120 150 230]+128)/383;patch([0 1 1 0],[0 0 1 1],c1);patch([0 1 1 1-e 1-e 0+e],[0 0 1 1-e 0+e 0+e],c2);patch([0 0 1 1-e 0+e 0+e],[0 1 1 1-e 1-e 0+e],c3);plot([0 1 1 0 0],[0 0 1 1 0]);disp('weights');
  "IW{3,2}(9,:)'" : Constant  Value=[-0.49701130325121045672176478547044098377227783203125;0.391882941495425851652356641352525912225246429443359375;-0.50614651186173542640744926757179200649261474609375;0.85085921387501972645850401022471487522125244140625;0.442862294766458275407927658307016827166080474853515625;-0.72958826753639882678470485188881866633892059326171875;0.5634242099819914972869128177990205585956573486328125;-0.483490427359628827108650739319273270666599273681640625;-0.2023989985885983333702142772381193935871124267578125;-0.57654221212125611462084862068877555429935455322265625]
      mask Display: e = 0.06;c1 = [120 150 230]/255;c2 = ([120 150 230]+0)/383;c3 = ([120 150 230]+128)/383;patch([0 1 1 0],[0 0 1 1],c1);patch([0 1 1 1-e 1-e 0+e],[0 0 1 1-e 0+e 0+e],c2);patch([0 0 1 1-e 0+e 0+e],[0 1 1 1-e 1-e 0+e],c3);plot([0 1 1 0 0],[0 0 1 1 0]);disp('weights');
  Mux : Mux  Inputs=10
      mask Display: e = 0.06;c1 = [120 150 230]/255;c2 = ([120 150 230]+0)/383;c3 = ([120 150 230]+128)/383;patch([0 1 1 0],[0 0 1 1],c1);patch([0 1 1 1-e 1-e 0+e],[0 0 1 1-e 0+e 0+e],c2);patch([0 0 1 1-e 0+e 0+e],[0 1 1 1-e 1-e 0+e],c3);plot([0 1 1 0 0],[0 0 1 1 0]);disp('Mux');
  dotprod{1..10} (10 alike) : neural/Weight Functions/dotprod
  "lz{3,2}" : Outport
      mask Display: e = 0.06;c1 = [120 230 180]/255;c2 = ([120 230 180]+0)/(256+128);c3 = ([120 230 180]+128)/(256+128);patch([0 1 1 0],[0 0 1 1],c1);patch([0 1 1 1-e 1-e 0+e],[0 0 1 1-e 0+e 0+e],c2);patch([0 0 1 1-e 0+e 0+e],[0 1 1 1-e 1-e 0+e],c3);plot([0 1 1 0 0],[0 0 1 1 0]);
  wires:
  "IW{3,2}(1,:)'"/1 -> dotprod1/1
  "ad{3,2}"/1 -> dotprod1/2, dotprod2/2, dotprod3/2, dotprod4/2, dotprod5/2, dotprod6/2, dotprod7/2, dotprod8/2, dotprod9/2, dotprod10/2
  dotprod1/1 -> Mux/1
  "IW{3,2}(2,:)'"/1 -> dotprod2/1
  dotprod2/1 -> Mux/2
  "IW{3,2}(3,:)'"/1 -> dotprod3/1
  dotprod3/1 -> Mux/3
  "IW{3,2}(4,:)'"/1 -> dotprod4/1
  dotprod4/1 -> Mux/4
  "IW{3,2}(5,:)'"/1 -> dotprod5/1
  dotprod5/1 -> Mux/5
  "IW{3,2}(6,:)'"/1 -> dotprod6/1
  dotprod6/1 -> Mux/6
  "IW{3,2}(7,:)'"/1 -> dotprod7/1
  dotprod7/1 -> Mux/7
  "IW{3,2}(8,:)'"/1 -> dotprod8/1
  dotprod8/1 -> Mux/8
  "IW{3,2}(9,:)'"/1 -> dotprod9/1
  dotprod9/1 -> Mux/9
  "IW{3,2}(10,:)'"/1 -> dotprod10/1
  dotprod10/1 -> Mux/10
  Mux/1 -> "lz{3,2}"/1

== system state_space_all_reduce_uio/Function Fitting Neural Network2/Layer 4/Delays 1 ==
  "p{4}" : Inport  PortDimensions=10  SampleTime=4e-05
      mask Display: e = 0.06;c1 = [120 230 180]/255;c2 = ([120 230 180]+0)/(256+128);c3 = ([120 230 180]+128)/(256+128);patch([0 1 1 0],[0 0 1 1],c1);patch([0 1 1 1-e 1-e 0+e],[0 0 1 1-e 0+e 0+e],c2);patch([0 0 1 1-e 0+e 0+e],[0 1 1 1-e 1-e 0+e],c3);plot([0 1 1 0 0],[0 0 1 1 0]);
  mux : Mux  Inputs=1
      mask Display: e = 0.06;c1 = [120 150 230]/255;c2 = ([120 150 230]+0)/383;c3 = ([120 150 230]+128)/383;patch([0 1 1 0],[0 0 1 1],c1);patch([0 1 1 1-e 1-e 0+e],[0 0 1 1-e 0+e 0+e],c2);patch([0 0 1 1-e 0+e 0+e],[0 1 1 1-e 1-e 0+e],c3);plot([0 1 1 0 0],[0 0 1 1 0]);disp('Mux')
  "pd{4,3}" : Outport
      mask Display: e = 0.06;c1 = [120 230 180]/255;c2 = ([120 230 180]+0)/(256+128);c3 = ([120 230 180]+128)/(256+128);patch([0 1 1 0],[0 0 1 1],c1);patch([0 1 1 1-e 1-e 0+e],[0 0 1 1-e 0+e 0+e],c2);patch([0 0 1 1-e 0+e 0+e],[0 1 1 1-e 1-e 0+e],c3);plot([0 1 1 0 0],[0 0 1 1 0]);
  wires:
  "p{4}"/1 -> mux/1
  mux/1 -> "pd{4,3}"/1

== system state_space_all_reduce_uio/Function Fitting Neural Network2/Layer 4/LW{4,3} ==
  "ad{4,3}" : Inport  PortDimensions=10  SampleTime=4e-05
      mask Display: e = 0.06;c1 = [120 230 180]/255;c2 = ([120 230 180]+0)/(256+128);c3 = ([120 230 180]+128)/(256+128);patch([0 1 1 0],[0 0 1 1],c1);patch([0 1 1 1-e 1-e 0+e],[0 0 1 1-e 0+e 0+e],c2);patch([0 0 1 1-e 0+e 0+e],[0 1 1 1-e 1-e 0+e],c3);plot([0 1 1 0 0],[0 0 1 1 0]);
  "IW{4,3}(1,:)'" : Constant  Value=[0.621771107646718501626992292585782706737518310546875;-0.7199192460133383431042375377728603780269622802734375;0.2322025582206237448446017879177816212177276611328125;-0.7360357762050584451429813270806334912776947021484375;0.176538768283716562823570939144701696932315826416015625;0.28319323992536660217211874623899348080158233642578125;-0.167248491530773979452106914322939701378345489501953125;-0.414367406120177250716807293429155834019184112548828125;0.435134289815036379156509838139754720032215118408203125;-0.90096724567177244313853634594124741852283477783203125]
      mask Display: e = 0.06;c1 = [120 150 230]/255;c2 = ([120 150 230]+0)/383;c3 = ([120 150 230]+128)/383;patch([0 1 1 0],[0 0 1 1],c1);patch([0 1 1 1-e 1-e 0+e],[0 0 1 1-e 0+e 0+e],c2);patch([0 0 1 1-e 0+e 0+e],[0 1 1 1-e 1-e 0+e],c3);plot([0 1 1 0 0],[0 0 1 1 0]);disp('weights');
  Mux : Mux  Inputs=1
      mask Display: e = 0.06;c1 = [120 150 230]/255;c2 = ([120 150 230]+0)/383;c3 = ([120 150 230]+128)/383;patch([0 1 1 0],[0 0 1 1],c1);patch([0 1 1 1-e 1-e 0+e],[0 0 1 1-e 0+e 0+e],c2);patch([0 0 1 1-e 0+e 0+e],[0 1 1 1-e 1-e 0+e],c3);plot([0 1 1 0 0],[0 0 1 1 0]);disp('Mux');
  dotprod1 : neural/Weight Functions/dotprod
  "lz{4,3}" : Outport
      mask Display: e = 0.06;c1 = [120 230 180]/255;c2 = ([120 230 180]+0)/(256+128);c3 = ([120 230 180]+128)/(256+128);patch([0 1 1 0],[0 0 1 1],c1);patch([0 1 1 1-e 1-e 0+e],[0 0 1 1-e 0+e 0+e],c2);patch([0 0 1 1-e 0+e 0+e],[0 1 1 1-e 1-e 0+e],c3);plot([0 1 1 0 0],[0 0 1 1 0]);
  wires:
  "IW{4,3}(1,:)'"/1 -> dotprod1/1
  "ad{4,3}"/1 -> dotprod1/2
  dotprod1/1 -> Mux/1
  Mux/1 -> "lz{4,3}"/1

== system state_space_all_reduce_uio/Function Fitting Neural Network3/Layer 1/Delays 1 ==
  "p{1}" : Inport  PortDimensions=44  SampleTime=4e-05
      mask Display: e = 0.06;c1 = [120 230 180]/255;c2 = ([120 230 180]+0)/(256+128);c3 = ([120 230 180]+128)/(256+128);patch([0 1 1 0],[0 0 1 1],c1);patch([0 1 1 1-e 1-e 0+e],[0 0 1 1-e 0+e 0+e],c2);patch([0 0 1 1-e 0+e 0+e],[0 1 1 1-e 1-e 0+e],c3);plot([0 1 1 0 0],[0 0 1 1 0]);
  mux : Mux  Inputs=1
      mask Display: e = 0.06;c1 = [120 150 230]/255;c2 = ([120 150 230]+0)/383;c3 = ([120 150 230]+128)/383;patch([0 1 1 0],[0 0 1 1],c1);patch([0 1 1 1-e 1-e 0+e],[0 0 1 1-e 0+e 0+e],c2);patch([0 0 1 1-e 0+e 0+e],[0 1 1 1-e 1-e 0+e],c3);plot([0 1 1 0 0],[0 0 1 1 0]);disp('Mux')
  "pd{1,1}" : Outport
      mask Display: e = 0.06;c1 = [120 230 180]/255;c2 = ([120 230 180]+0)/(256+128);c3 = ([120 230 180]+128)/(256+128);patch([0 1 1 0],[0 0 1 1],c1);patch([0 1 1 1-e 1-e 0+e],[0 0 1 1-e 0+e 0+e],c2);patch([0 0 1 1-e 0+e 0+e],[0 1 1 1-e 1-e 0+e],c3);plot([0 1 1 0 0],[0 0 1 1 0]);
  wires:
  "p{1}"/1 -> mux/1
  mux/1 -> "pd{1,1}"/1
